simulink model "motor"  (R2020b)
settings: Solver=VariableStepAuto  StartTime=0.0  StopTime=10.0  RelTol=1e-3
settings Model: Creator=leo7s  LastModifiedBy=leo7s

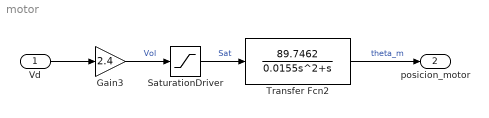
== system motor ==
  Vd : Inport
  Gain3 : Gain  Gain=2.4
  SaturationDriver : Saturate  UpperLimit=12  LowerLimit=0
  Transfer Fcn2 : TransferFcn  Numerator=[89.7462]  Denominator=[0.0155 1 0]
  posicion_motor : Outport  Port=2
  wires:
  Vd/1 -> Gain3/1
  Transfer Fcn2/1 -> posicion_motor/1  "theta_m"
  Gain3/1 -> SaturationDriver/1  "Vol"
  SaturationDriver/1 -> Transfer Fcn2/1  "Sat"
